simulink model "Q1"  (R2018a)
settings: Solver=VariableStepAuto  StartTime=0.0  StopTime=18  RelTol=1e-3
libraries: simulink x1
settings Model: Creator=Rodrigo  LastModifiedBy=Rodrigo

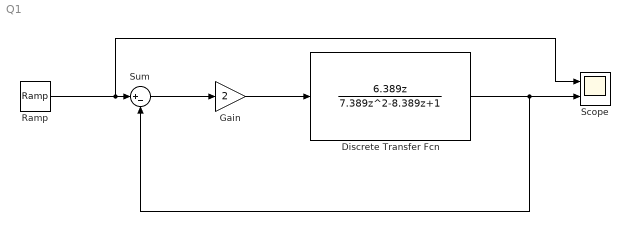
== system Q1 ==
  Discrete Transfer Fcn : DiscreteTransferFcn  Numerator=[6.389 0]  Denominator=[7.389 -8.389 1]  SampleTime=2
  Gain : Gain  Gain=2
  Ramp : simulink/Sources/Ramp  slope=1  start=0  InitialOutput=0
  Scope : Scope  NumInputPorts=2
  Sum : Sum  Inputs=|+-
  wires:
  Discrete Transfer Fcn/1 -> Sum/2, Scope/2
  Gain/1 -> Discrete Transfer Fcn/1
  Sum/1 -> Gain/1
  Ramp/1 -> Scope/1, Sum/1
